simulink model "SkidSteerKinematics"  (R2026a)
settings: Solver=FixedStepDiscrete  StopTime=10  FixedStep=0.02
model workspace (MAT data in the model file):
  P.wheel_radius = 0.1651
  P.wheel_separation = 0.617
  P.wheel_separation_multiplier = 1.659
  P.wheel_joint_velocity_limit = 10.958
  P.diff_drive_update_rate = 50
  P.dt = 0.02
Description:
  | As-built skid-steer kinematics (rover_controller diff_drive). Generated by scripts/build_skid_steer.m.
settings Model: Creator=potlo  LastModifiedBy=potlo
settings DataIOCC: LoadExternalInput=on

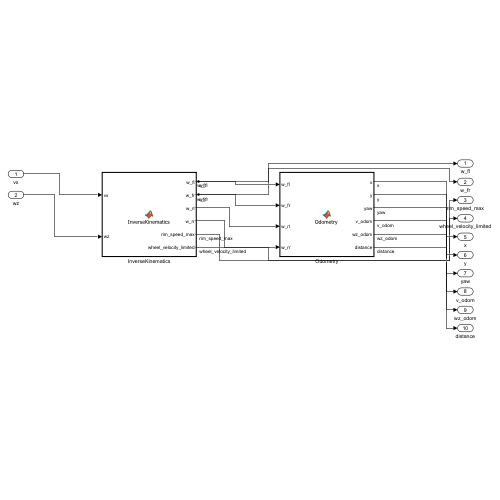
[thumbnail: Simulink's stored preview of the top-level diagram]
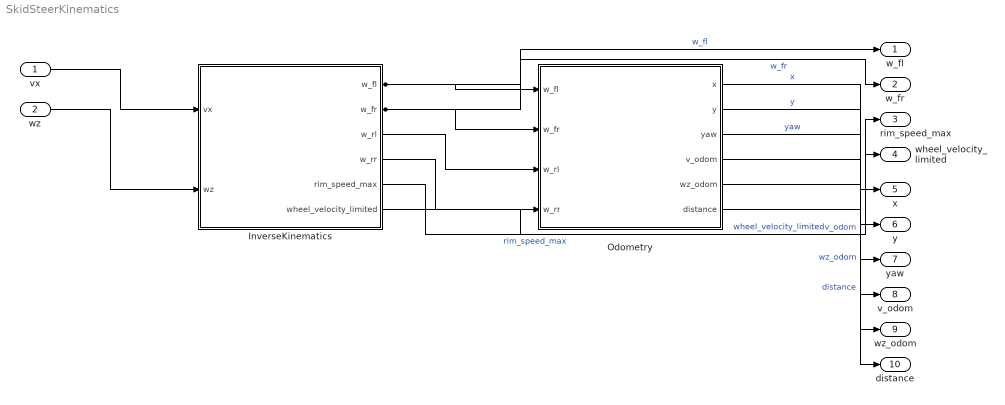
== system SkidSteerKinematics ==
  vx : Inport  Interpolate=off
  wz : Inport  Port=2  Interpolate=off
  InverseKinematics : MATLAB Function  TreatAsAtomicUnit=on
  Odometry : MATLAB Function  TreatAsAtomicUnit=on
  w_fl : Outport
  w_fr : Outport  Port=2
  rim_speed_max : Outport  Port=3
  wheel_velocity_limited : Outport  Port=4
  x : Outport  Port=5
  y : Outport  Port=6
  yaw : Outport  Port=7
  v_odom : Outport  Port=8
  wz_odom : Outport  Port=9
  distance : Outport  Port=10
  wires:
  InverseKinematics/1(w_fl) -> Odometry/1(w_fl), w_fl/1  "w_fl"
  InverseKinematics/2(w_fr) -> Odometry/2(w_fr), w_fr/1  "w_fr"
  InverseKinematics/3(w_rl) -> Odometry/3(w_rl)
  InverseKinematics/4(w_rr) -> Odometry/4(w_rr)
  vx/1 -> InverseKinematics/1(vx)
  wz/1 -> InverseKinematics/2(wz)
  InverseKinematics/5(rim_speed_max) -> rim_speed_max/1  "rim_speed_max"
  InverseKinematics/6(wheel_velocity_limited) -> wheel_velocity_limited/1  "wheel_velocity_limited"
  Odometry/1(x) -> x/1  "x"
  Odometry/2(y) -> y/1  "y"
  Odometry/3(yaw) -> yaw/1  "yaw"
  Odometry/4(v_odom) -> v_odom/1  "v_odom"
  Odometry/5(wz_odom) -> wz_odom/1  "wz_odom"
  Odometry/6(distance) -> distance/1  "distance"

== matlab function SkidSteerKinematics/Odometry ==
  data: x output; w_fl input; y output; w_fr input; w_rl input; w_rr input; yaw output; v_odom output; wz_odom output; distance output; P parameter
function [x, y, yaw, v_odom, wz_odom, distance] = Odometry(w_fl, w_fr, w_rl, w_rr, P)
persistent px py pyaw pdist
if isempty(px), px = 0; py = 0; pyaw = 0; pdist = 0; end
track = P.wheel_separation * P.wheel_separation_multiplier;
w_left = (w_fl + w_rl) / 2; w_right = (w_fr + w_rr) / 2;
v_odom = P.wheel_radius * (w_left + w_right) / 2;
wz_odom = P.wheel_radius * (w_right - w_left) / track;
px = px + v_odom * cos(pyaw + wz_odom * P.dt / 2) * P.dt;
py = py + v_odom * sin(pyaw + wz_odom * P.dt / 2) * P.dt;
pyaw = pyaw + wz_odom * P.dt;
pdist = pdist + abs(v_odom) * P.dt;
x = px; y = py; yaw = pyaw; distance = pdist;

== matlab function SkidSteerKinematics/InverseKinematics ==
  data: vx input; w_fl output; wz input; w_fr output; w_rl output; w_rr output; rim_speed_max output; wheel_velocity_limited output; P parameter
function [w_fl, w_fr, w_rl, w_rr, rim_speed_max, wheel_velocity_limited] = InverseKinematics(vx, wz, P)
track = P.wheel_separation * P.wheel_separation_multiplier;
w_left = (vx - wz * track / 2) / P.wheel_radius;
w_right = (vx + wz * track / 2) / P.wheel_radius;
w_fl = w_left; w_rl = w_left; w_fr = w_right; w_rr = w_right;
rim_speed_max = max(abs([w_left w_right])) * P.wheel_radius;
wheel_velocity_limited = double(max(abs([w_left w_right])) > P.wheel_joint_velocity_limit);
